simulink model "i2c_example"  (R2025a)
settings: Solver=FixedStepDiscrete  StartTime=0.0  StopTime=Inf  FixedStep=Auto  RelTol=1e-3  EnableMultiTasking=on
libraries: c280xlib x8, simulink x8, demo_controls x1
settings Model: SimulationMode=external  ExtModeTrigDuration=8  Creator=The MathWorks, Inc.  LastModifiedBy=Sindi
settings SolverCC: AlgebraicLoopSolver=TrustRegion
settings DataIOCC: LimitDataPoints=on  SaveFormat=Array  SaveOutput=off  SaveTime=off  ReturnWorkspaceOutputs=off
settings OptimizationCC: BlockReduction=off  ConditionallyExecuteInputs=off  DefaultUnderspecifiedDataType=single  OptimizeBlockIOStorage=off  BufferReuse=off  GlobalBufferReuse=off  ExpressionFolding=off  ExpressionDepthLimit=2147483647.0  LocalBlockOutputs=off  InitFltsAndDblsToZero=on  LifeSpan=Inf  MaxStackSize=1024  EfficientTunableParamExpr=on
settings DebuggingCC: UnderspecifiedInitializationDetection=Classic  MergeDetectMultiDrivingBlocksExec=none  SolverPrmCheckMsg=warning  InheritedTsInSrcMsg=none  FcnCallInpInsideContextMsg=warning  UnconnectedInputMsg=warning  UnconnectedOutputMsg=warning  UnconnectedLineMsg=warning  AllowSymbolicDim=off  StateNameClashWarn=warning  SFUnexpectedBacktrackingDiag=warning  SFNoUnconditionalDefaultTransitionDiag=warning  SFExecutionAtInitializationDiag=none  ArithmeticOperatorsInVariantConditions=warning
settings HardwareCC: ProdBitPerChar=16.0  ProdBitPerInt=16.0  ProdBitPerPointer=32.0  ProdBitPerSizeT=32.0  ProdBitPerPtrDiffT=32.0  ProdLargestAtomicInteger=Integer  ProdLargestAtomicFloat=None  ProdWordSize=16.0  ProdLongLongMode=on  ProdHWDeviceType=Texas Instruments->C2000  TargetBitPerChar=16.0  TargetBitPerInt=16.0  TargetBitPerPointer=16.0  TargetIntDivRoundTo=Zero  TargetEndianess=LittleEndian  TargetWordSize=16.0  TargetHWDeviceType=TI C2000  HardwareBoardFeatureSet=SoCBlockset
settings ModelReferenceCC: EnableRefExpFcnMdlSchedulingChecks=on  ModelReferenceNumInstancesAllowed=Single  PropagateSignalLabelsOutOfModel=off
settings SFSimCC: SimUseLocalCustomCode=off  SimParseCustomCode=off  CustomCodeUndefinedFunction=UseInterfaceOnly
settings RTWCC: SystemTargetFile=ert.tlc  HardwareBoard=TI Delfino F28379D LaunchPad  TemplateMakefile=ert_default_tmf  RTWUseLocalCustomCode=off  Toolchain=Texas Instruments Code Composer Studio (C2000)  CodeProfilingSaveOptions=MetricsOnly  GPUComputeCapability=3.5  DLArmComputeVersion=19.05  Description=Embedded Coder
settings CodeAppCC: IgnoreCustomStorageClasses=off  CustomSymbolStrType=$N$R$M  StateflowObjectComments=on  InternalIdentifier=Classic
settings ERTTargetCC: ExtModeTransport=4.0  ExtModeAutomaticAllocSize=off  ExtModeStaticAllocSize=10000.0  InlinedParameterPlacement=Hierarchical  ConvertIfToSwitch=off  SuppressUnreachableDefaultCases=off  DynamicArrayContainerType=coder::array  CodeReplacementLibrary=TI C28x  MultiwordLength=2048.0  SubcomponentCodeInterfacePackaging=Nonreusable function
settings ConfigComp: CovMetricSettings=dw  CovSaveCumulativeToWorkspaceVar=on  CovSaveSingleToWorkspaceVar=on  CovExternalEMLEnable=off  CovSFcnEnable=off

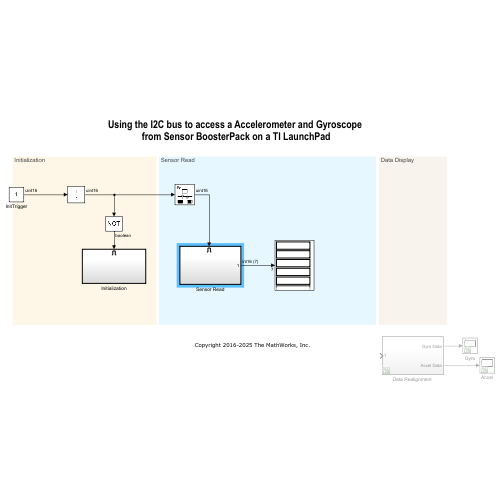
[thumbnail: Simulink's stored preview of the top-level diagram]
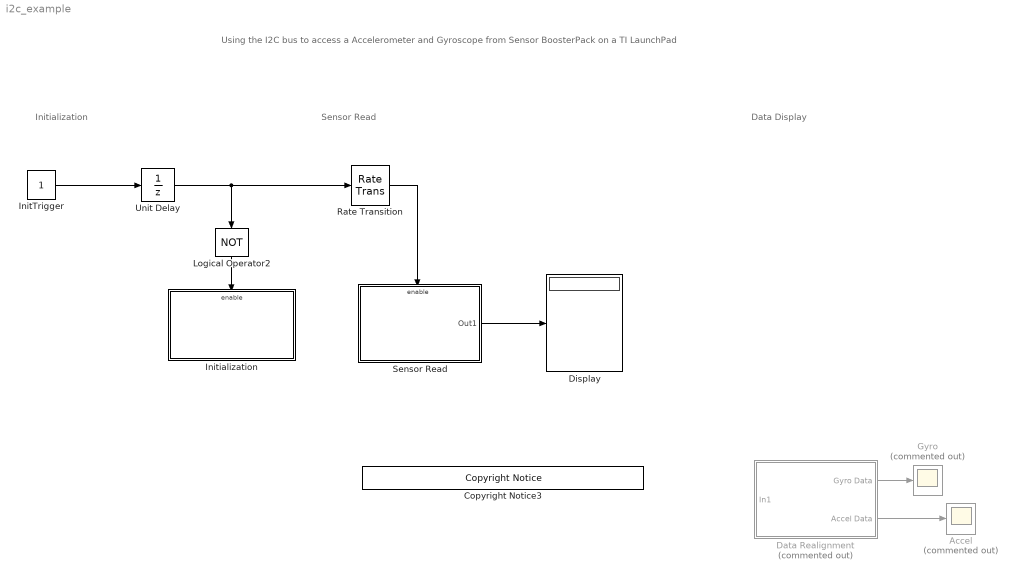
== system i2c_example ==
  note: Using the I2C bus to access a Accelerometer and Gyroscope
      | from Sensor BoosterPack on a TI LaunchPad
  note: Initialization
  note: Data Display
  note: Sensor Read
  Accel : Scope  Commented=on
      settings: TimeUnits=Metric (based on Time Span)  ActiveDisplayYMinimum=-16899  ActiveDisplayYMaximum=23871  YLabel=Amplitude  DataLoggingSaveFormat=Array
  Copyright Notice3 : demo_controls/Copyright Notice  year=2016  prod=tic2000
  "Data Realignment " : Subsystem  Commented=on
  Display : Display
  Gyro : Scope  Commented=on
      settings: TimeUnits=Metric (based on Time Span)  ActiveDisplayYMinimum=-8144.75  ActiveDisplayYMaximum=9082.75  YLabel=Amplitude  DataLoggingVariableName=ScopeData2  DataLoggingSaveFormat=Array
  InitTrigger : Constant  Priority=10  OutDataTypeStr=uint16  SampleTime=0.1
  Initialization : Subsystem
  Logical Operator2 : Logic  Operator=NOT  AllPortsSameDT=off  OutDataTypeStr=boolean
  Rate Transition : RateTransition  OutPortSampleTime=1e-3
  Sensor Read : Subsystem  Priority=10  TreatAsAtomicUnit=on
  Unit Delay : UnitDelay  SampleTime=-1  HasFrameUpgradeWarning=on
  wires:
  Unit Delay/1 -> Rate Transition/1, Logical Operator2/1
  "Data Realignment "/1(Gyro Data) -> Gyro/1
  "Data Realignment "/2(Accel Data) -> Accel/1
  Logical Operator2/1 -> Initialization/Enable
  Rate Transition/1 -> Sensor Read/Enable
  InitTrigger/1 -> Unit Delay/1
  Sensor Read/1(Out1) -> Display/1

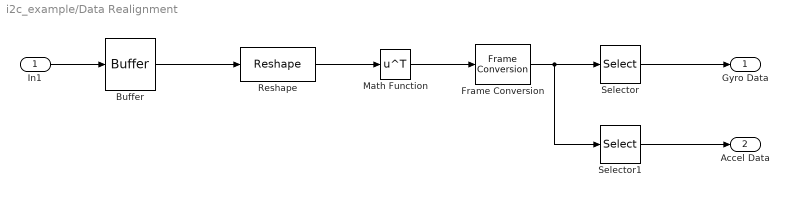
== system i2c_example/Data Realignment  ==
  In1 : Inport
  Buffer : Buffer  N=30*6
  Frame Conversion : FrameConversion
  Math Function : Math  Operator=transpose  SignedPower=on
  Reshape : Reshape  OutputDimensionality=Customize  OutputDimensions=[6,30]
  Selector : Selector  NumberOfDimensions=2  InputPortWidth=3  IndexOptions=Index vector (dialog),Starting index (dialog)  Indices=1:30,1  OutputSizes=1,3
  Selector1 : Selector  NumberOfDimensions=2  InputPortWidth=3  IndexOptions=Index vector (dialog),Starting index (dialog)  Indices=1:30,4  OutputSizes=1,3
  Gyro Data : Outport  VectorParamsAs1DForOutWhenUnconnected=off
  Accel Data : Outport  Port=2  VectorParamsAs1DForOutWhenUnconnected=off
  wires:
  In1/1 -> Buffer/1
  Reshape/1 -> Math Function/1
  Buffer/1 -> Reshape/1
  Frame Conversion/1 -> Selector1/1, Selector/1
  Math Function/1 -> Frame Conversion/1
  Selector/1 -> Gyro Data/1
  Selector1/1 -> Accel Data/1

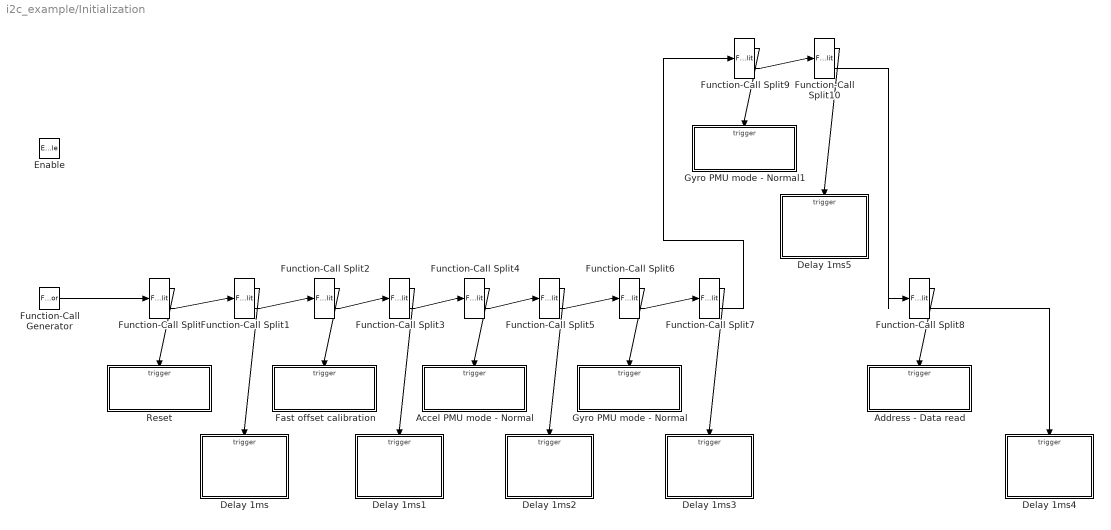
== system i2c_example/Initialization ==
  Enable : EnablePort
  Accel PMU mode - Normal : Subsystem  TreatAsAtomicUnit=on
  Address - Data read : Subsystem  TreatAsAtomicUnit=on
  Delay 1ms : Subsystem  TreatAsAtomicUnit=on
  Delay 1ms1 : Subsystem  TreatAsAtomicUnit=on
  Delay 1ms2 : Subsystem  TreatAsAtomicUnit=on
  Delay 1ms3 : Subsystem  TreatAsAtomicUnit=on
  Delay 1ms4 : Subsystem  TreatAsAtomicUnit=on
  Delay 1ms5 : Subsystem  TreatAsAtomicUnit=on
  Fast offset calibration : Subsystem  TreatAsAtomicUnit=on
  Function-Call Generator : FunctionCallGenerator  SampleTime=-1
  Function-Call Split{,1..10} (11 alike) : FunctionCallSplit  NumOutputPorts=2
  Gyro PMU mode - Normal : Subsystem  TreatAsAtomicUnit=on
  Gyro PMU mode - Normal1 : Subsystem  TreatAsAtomicUnit=on
  Reset : Subsystem  TreatAsAtomicUnit=on
  wires:
  Function-Call Split4/1 -> Accel PMU mode - Normal/Trigger
  Function-Call Split3/2 -> Function-Call Split4/1
  Function-Call Split1/1 -> Delay 1ms/Trigger
  Function-Call Split2/1 -> Fast offset calibration/Trigger
  Function-Call Split5/2 -> Function-Call Split6/1
  Function-Call Split/2 -> Function-Call Split1/1
  Function-Call Split1/2 -> Function-Call Split2/1
  Function-Call Split8/1 -> Address - Data read/Trigger
  Function-Call Split6/2 -> Function-Call Split7/1
  Function-Call Split4/2 -> Function-Call Split5/1
  Function-Call Generator/1 -> Function-Call Split/1
  Function-Call Split7/1 -> Delay 1ms3/Trigger
  Function-Call Split5/1 -> Delay 1ms2/Trigger
  Function-Call Split/1 -> Reset/Trigger
  Function-Call Split3/1 -> Delay 1ms1/Trigger
  Function-Call Split8/2 -> Delay 1ms4/Trigger
  Function-Call Split6/1 -> Gyro PMU mode - Normal/Trigger
  Function-Call Split2/2 -> Function-Call Split3/1
  Function-Call Split9/2 -> Function-Call Split10/1
  Function-Call Split10/1 -> Delay 1ms5/Trigger
  Function-Call Split9/1 -> Gyro PMU mode - Normal1/Trigger
  Function-Call Split7/2 -> Function-Call Split9/1
  Function-Call Split10/2 -> Function-Call Split8/1

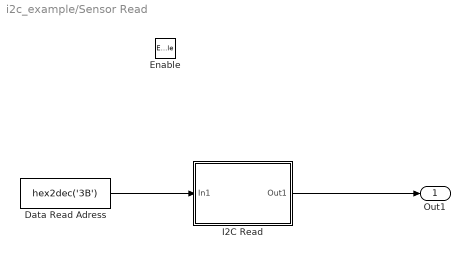
== system i2c_example/Sensor Read ==
  Enable : EnablePort
  Data Read Adress : Constant  Priority=10  Value=hex2dec('3B')  OutDataTypeStr=uint8  SampleTime=-1
  I2C Read : Subsystem
  Out1 : Outport
  wires:
  Data Read Adress/1 -> I2C Read/1(In1)
  I2C Read/1(Out1) -> Out1/1

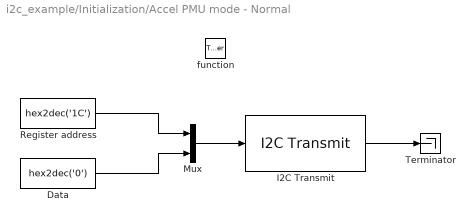
== system i2c_example/Initialization/Accel PMU mode - Normal ==
  function : TriggerPort  TriggerType=function-call  VariantControl=Variant
  Data : Constant  Value=hex2dec('0')  OutDataTypeStr=uint8  SampleTime=-1
  I2C Transmit : c280xlib/I2C Transmit  selectModule=I2C_A  addrFormat=7-Bit addressing  saSource=Specify via dialog  SAR=104  bitCount=8  STP=on  RM=off  STR=on
  Mux : Mux  Inputs=2
  Register address : Constant  Value=hex2dec('1C')  OutDataTypeStr=uint8  SampleTime=-1
  Terminator : Terminator
  wires:
  Register address/1 -> Mux/1
  Data/1 -> Mux/2
  I2C Transmit/1 -> Terminator/1
  Mux/1 -> I2C Transmit/1

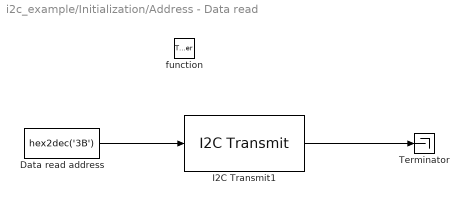
== system i2c_example/Initialization/Address - Data read ==
  function : TriggerPort  TriggerType=function-call  VariantControl=Variant
  Data read address : Constant  Value=hex2dec('3B')  OutDataTypeStr=uint8  SampleTime=-1
  I2C Transmit1 : c280xlib/I2C Transmit  selectModule=I2C_A  addrFormat=7-Bit addressing  saSource=Specify via dialog  SAR=104  bitCount=8  STP=off  RM=off  STR=on
  Terminator : Terminator
  wires:
  Data read address/1 -> I2C Transmit1/1
  I2C Transmit1/1 -> Terminator/1

== system i2c_example/Initialization/Delay 1ms ==
  function : TriggerPort  TriggerType=function-call  VariantControl=Variant
  System Outputs : Subsystem  mask(System Outputs){ShowInLibBrowser=0}
      mask prompts: ShowInLibBrowser "Simulink:masks:CustCodeMaskParam1_MP"
      settings: CopyFcn=cccopyfcn(gcb)  OpenFcn=ccopenfcn('System Outputs Function')
      mask Help: eval('feval(''rtwprivate'',''rtwhelpview'',''rtw_sys_outputs_block'')');
      mask Display: disp('System\nOutputs');

== system i2c_example/Initialization/Delay 1ms1 ==
  function : TriggerPort  TriggerType=function-call  VariantControl=Variant
  System Outputs : Subsystem  mask(System Outputs){ShowInLibBrowser=0}
      mask prompts: ShowInLibBrowser "Simulink:masks:CustCodeMaskParam1_MP"
      settings: CopyFcn=cccopyfcn(gcb)  OpenFcn=ccopenfcn('System Outputs Function')
      mask Help: eval('feval(''rtwprivate'',''rtwhelpview'',''rtw_sys_outputs_block'')');
      mask Display: disp('System\nOutputs');

== system i2c_example/Initialization/Delay 1ms2 ==
  function : TriggerPort  TriggerType=function-call  VariantControl=Variant
  System Outputs : Subsystem  mask(System Outputs){ShowInLibBrowser=0}
      mask prompts: ShowInLibBrowser "Simulink:masks:CustCodeMaskParam1_MP"
      settings: CopyFcn=cccopyfcn(gcb)  OpenFcn=ccopenfcn('System Outputs Function')
      mask Help: eval('feval(''rtwprivate'',''rtwhelpview'',''rtw_sys_outputs_block'')');
      mask Display: disp('System\nOutputs');

== system i2c_example/Initialization/Delay 1ms3 ==
  function : TriggerPort  TriggerType=function-call  VariantControl=Variant
  System Outputs : Subsystem  mask(System Outputs){ShowInLibBrowser=0}
      mask prompts: ShowInLibBrowser "Simulink:masks:CustCodeMaskParam1_MP"
      settings: CopyFcn=cccopyfcn(gcb)  OpenFcn=ccopenfcn('System Outputs Function')
      mask Help: eval('feval(''rtwprivate'',''rtwhelpview'',''rtw_sys_outputs_block'')');
      mask Display: disp('System\nOutputs');

== system i2c_example/Initialization/Delay 1ms4 ==
  function : TriggerPort  TriggerType=function-call  VariantControl=Variant
  System Outputs : Subsystem  mask(System Outputs){ShowInLibBrowser=0}
      mask prompts: ShowInLibBrowser "Simulink:masks:CustCodeMaskParam1_MP"
      settings: CopyFcn=cccopyfcn(gcb)  OpenFcn=ccopenfcn('System Outputs Function')
      mask Help: eval('feval(''rtwprivate'',''rtwhelpview'',''rtw_sys_outputs_block'')');
      mask Display: disp('System\nOutputs');

== system i2c_example/Initialization/Delay 1ms5 ==
  function : TriggerPort  TriggerType=function-call  VariantControl=Variant
  System Outputs : Subsystem  mask(System Outputs){ShowInLibBrowser=0}
      mask prompts: ShowInLibBrowser "Simulink:masks:CustCodeMaskParam1_MP"
      settings: CopyFcn=cccopyfcn(gcb)  OpenFcn=ccopenfcn('System Outputs Function')
      mask Help: eval('feval(''rtwprivate'',''rtwhelpview'',''rtw_sys_outputs_block'')');
      mask Display: disp('System\nOutputs');

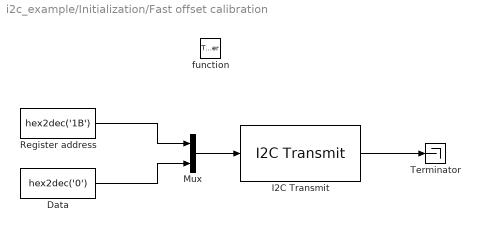
== system i2c_example/Initialization/Fast offset calibration ==
  function : TriggerPort  TriggerType=function-call  VariantControl=Variant
  Data : Constant  Value=hex2dec('0')  OutDataTypeStr=uint8  SampleTime=-1
  I2C Transmit : c280xlib/I2C Transmit  selectModule=I2C_A  addrFormat=7-Bit addressing  saSource=Specify via dialog  SAR=104  bitCount=8  STP=on  RM=off  STR=on
  Mux : Mux  Inputs=2
  Register address : Constant  Value=hex2dec('1B')  OutDataTypeStr=uint8  SampleTime=-1
  Terminator : Terminator
  wires:
  Data/1 -> Mux/2
  I2C Transmit/1 -> Terminator/1
  Mux/1 -> I2C Transmit/1
  Register address/1 -> Mux/1

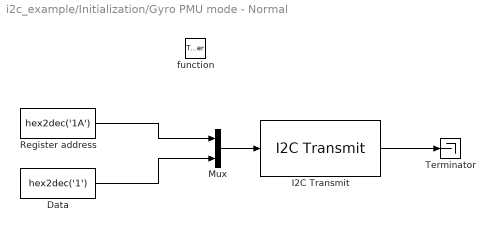
== system i2c_example/Initialization/Gyro PMU mode - Normal ==
  function : TriggerPort  TriggerType=function-call  VariantControl=Variant
  Data : Constant  Value=hex2dec('1')  OutDataTypeStr=uint8  SampleTime=-1
  I2C Transmit : c280xlib/I2C Transmit  selectModule=I2C_A  addrFormat=7-Bit addressing  saSource=Specify via dialog  SAR=104  bitCount=8  STP=on  RM=off  STR=on
  Mux : Mux  Inputs=2
  Register address : Constant  Value=hex2dec('1A')  OutDataTypeStr=uint8  SampleTime=-1
  Terminator : Terminator
  wires:
  I2C Transmit/1 -> Terminator/1
  Mux/1 -> I2C Transmit/1
  Register address/1 -> Mux/1
  Data/1 -> Mux/2

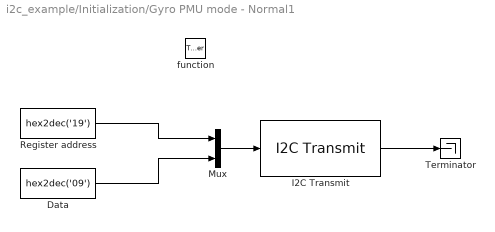
== system i2c_example/Initialization/Gyro PMU mode - Normal1 ==
  function : TriggerPort  TriggerType=function-call  VariantControl=Variant
  Data : Constant  Value=hex2dec('09')  OutDataTypeStr=uint8  SampleTime=-1
  I2C Transmit : c280xlib/I2C Transmit  selectModule=I2C_A  addrFormat=7-Bit addressing  saSource=Specify via dialog  SAR=104  bitCount=8  STP=on  RM=off  STR=on
  Mux : Mux  Inputs=2
  Register address : Constant  Value=hex2dec('19')  OutDataTypeStr=uint8  SampleTime=-1
  Terminator : Terminator
  wires:
  I2C Transmit/1 -> Terminator/1
  Mux/1 -> I2C Transmit/1
  Register address/1 -> Mux/1
  Data/1 -> Mux/2

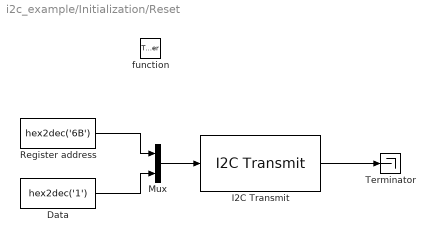
== system i2c_example/Initialization/Reset ==
  function : TriggerPort  TriggerType=function-call  VariantControl=Variant
  Data : Constant  Value=hex2dec('1')  OutDataTypeStr=uint8  SampleTime=-1
  I2C Transmit : c280xlib/I2C Transmit  selectModule=I2C_A  addrFormat=7-Bit addressing  saSource=Specify via dialog  SAR=104  bitCount=8  STP=on  RM=off  STR=on
  Mux : Mux  Inputs=2
  Register address : Constant  Value=hex2dec('6B')  OutDataTypeStr=uint8  SampleTime=-1
  Terminator : Terminator
  wires:
  Data/1 -> Mux/2
  Register address/1 -> Mux/1
  I2C Transmit/1 -> Terminator/1
  Mux/1 -> I2C Transmit/1

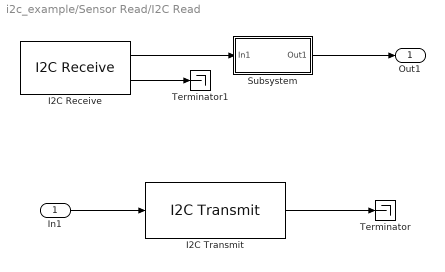
== system i2c_example/Sensor Read/I2C Read ==
  In1 : Inport
  I2C Receive : c280xlib/I2C Receive  Priority=10  selectModule=I2C_A  addrFormat=7-Bit addressing  saSource=Specify via dialog  SAR=104  bitCount=8  dataLength=14  initValue=0  NACK=off  STP=on  STR=on  sampleTime=-1  dataType=uint8
  I2C Transmit : c280xlib/I2C Transmit  Priority=20  selectModule=I2C_A  addrFormat=7-Bit addressing  saSource=Specify via dialog  SAR=104  bitCount=8  STP=off  RM=off  STR=on
  Subsystem : Subsystem
  Terminator : Terminator
  Terminator1 : Terminator
  Out1 : Outport  VectorParamsAs1DForOutWhenUnconnected=off
  wires:
  In1/1 -> I2C Transmit/1
  I2C Receive/1 -> Subsystem/1(In1)
  I2C Receive/2 -> Terminator1/1
  Subsystem/1(Out1) -> Out1/1
  I2C Transmit/1 -> Terminator/1

== system i2c_example/Initialization/Delay 1ms/System Outputs ==

== system i2c_example/Initialization/Delay 1ms1/System Outputs ==

== system i2c_example/Initialization/Delay 1ms2/System Outputs ==

== system i2c_example/Initialization/Delay 1ms3/System Outputs ==

== system i2c_example/Initialization/Delay 1ms4/System Outputs ==

== system i2c_example/Initialization/Delay 1ms5/System Outputs ==

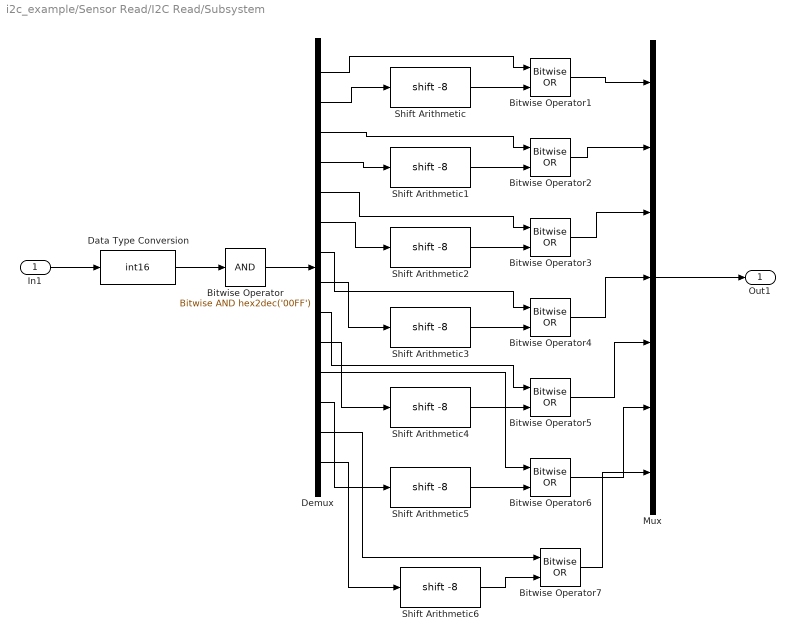
== system i2c_example/Sensor Read/I2C Read/Subsystem ==
  In1 : Inport
  Bitwise Operator : simulink/Logic and Bit Operations/Bitwise Operator  logicop=AND  UseBitMask=on  BitMask=hex2dec('00FF')  BitMaskRealWorld=Stored Integer
  Bitwise Operator{1..7} (7 alike) : simulink/Logic and Bit Operations/Bitwise Operator  logicop=OR  UseBitMask=off  NumInputPorts=2  BitMask=bin2dec('11011001')  BitMaskRealWorld=Stored Integer
  Data Type Conversion : DataTypeConversion  OutDataTypeStr=int16  ConvertRealWorld=Stored Integer (SI)  SaturateOnIntegerOverflow=off  RndMeth=Floor
  Demux : Demux  Outputs=14
  Mux : Mux  Inputs=7
  Shift Arithmetic{,1..6} (7 alike) : ArithShift  BitShiftNumber=-8
  Out1 : Outport  VectorParamsAs1DForOutWhenUnconnected=off
  wires:
  In1/1 -> Data Type Conversion/1
  Data Type Conversion/1 -> Bitwise Operator/1
  Mux/1 -> Out1/1
  Bitwise Operator/1 -> Demux/1
  Bitwise Operator4/1 -> Mux/4
  Bitwise Operator5/1 -> Mux/5
  Bitwise Operator3/1 -> Mux/3
  Bitwise Operator6/1 -> Mux/6
  Bitwise Operator1/1 -> Mux/1
  Bitwise Operator2/1 -> Mux/2
  Demux/1 -> Bitwise Operator1/1
  Demux/2 -> Shift Arithmetic/1
  Shift Arithmetic/1 -> Bitwise Operator1/2
  Demux/3 -> Bitwise Operator2/1
  Demux/4 -> Shift Arithmetic1/1
  Shift Arithmetic1/1 -> Bitwise Operator2/2
  Demux/5 -> Bitwise Operator3/1
  Shift Arithmetic2/1 -> Bitwise Operator3/2
  Demux/6 -> Shift Arithmetic2/1
  Demux/7 -> Bitwise Operator4/1
  Demux/8 -> Shift Arithmetic3/1
  Demux/9 -> Bitwise Operator5/1
  Demux/10 -> Shift Arithmetic4/1
  Demux/11 -> Bitwise Operator6/1
  Demux/12 -> Shift Arithmetic5/1
  Shift Arithmetic3/1 -> Bitwise Operator4/2
  Shift Arithmetic4/1 -> Bitwise Operator5/2
  Shift Arithmetic5/1 -> Bitwise Operator6/2
  Bitwise Operator7/1 -> Mux/7
  Shift Arithmetic6/1 -> Bitwise Operator7/2
  Demux/13 -> Bitwise Operator7/1
  Demux/14 -> Shift Arithmetic6/1
